simulink subsystem "EKF_IMU_GPS_3DoF"  (R2024b)
settings: Solver=VariableStepAuto  StartTime=0.0  StopTime=10.0  RelTol=1e-3
undefined symbols (not defined in the file or in its folder): filter_update_time, fractalcoef, lla_ref, u0, x0
libraries: sharedTrackingLibrary x1, sensorgpslib x1, mspsensorlib x1
settings Model: Creator=thatf  LastModifiedBy=thatf

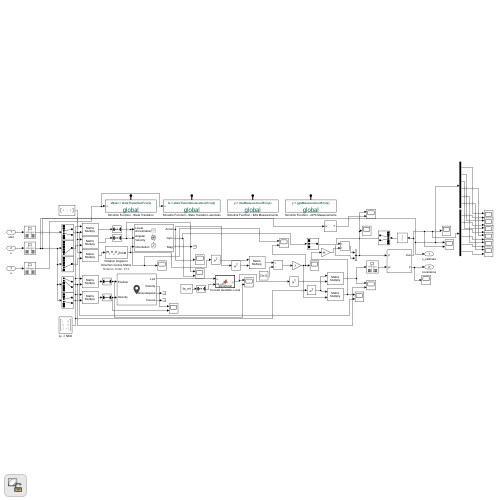
[thumbnail: Simulink's stored preview of the top-level diagram]
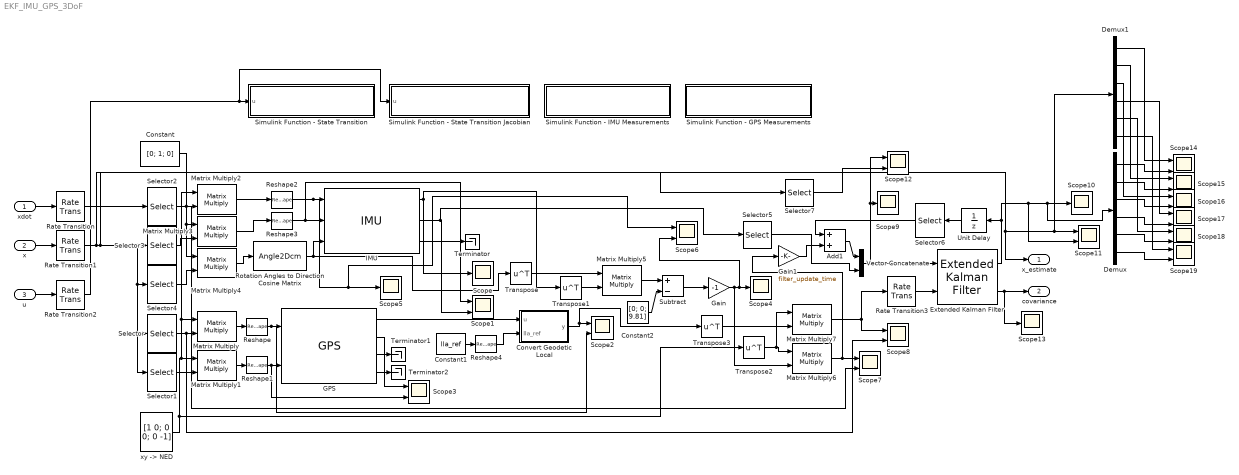
== system EKF_IMU_GPS_3DoF ==
  xdot : Inport
  x : Inport  Port=2
  u : Inport  Port=3
  Add1 : Sum
  Constant : Constant  Value=[0; 1; 0]
  Constant1 : Constant  Value=lla_ref
  Constant2 : Constant  Value=[0; 0; 9.81]
  Convert Geodetic Local : MATLAB Function  TreatAsAtomicUnit=on
  Demux : Demux  Outputs=6
  Demux1 : Demux  Outputs=6
  Extended Kalman Filter : sharedTrackingLibrary/Extended Kalman Filter  StateTransitionFcn=stateTransitionFcn  HasStateTransitionJacobianFcn=on  StateTransitionJacobianFcn=stateTransitionJacobianFcn  HasAdditiveProcessNoise=Additive  ProcessNoise=eye(6)*0.1  HasTimeVaryingProcessNoise=off  HasStateTransitionFcnExtraArgument=0  InitialState=x0'  InitialStateCovariance=eye(6)*0.1  MeasurementFcn1=imuMeasurementFcn  HasMeasurementJacobianFcn1=off  HasMeasurementEnablePort1=off  HasAdditiveMeasurementNoise1=Additive  MeasurementNoise1=[0.001;0.001;0.0001]  HasTimeVaryingMeasurementNoise1=off  HasMeasurementFcnExtraArgument1=0  HasMeasurementWrapping1=off  MeasurementFcn2=gpsMeasurementFcn  HasMeasurementJacobianFcn2=off  HasMeasurementEnablePort2=off  HasAdditiveMeasurementNoise2=Additive  MeasurementNoise2=[0.0005;.0001]  HasTimeVaryingMeasurementNoise2=off  HasMeasurementFcnExtraArgument2=0  HasMeasurementWrapping2=off  MeasurementFcn3=myMeasurementFcn  HasMeasurementJacobianFcn3=off  HasMeasurementEnablePort3=off  HasAdditiveMeasurementNoise3=Additive  MeasurementNoise3=1  HasTimeVaryingMeasurementNoise3=off  HasMeasurementFcnExtraArgument3=0  HasMeasurementWrapping3=off  MeasurementFcn4=myMeasurementFcn  HasMeasurementJacobianFcn4=off  HasMeasurementEnablePort4=off  HasAdditiveMeasurementNoise4=Additive  MeasurementNoise4=1  HasTimeVaryingMeasurementNoise4=off  HasMeasurementFcnExtraArgument4=0  HasMeasurementWrapping4=off  MeasurementFcn5=myMeasurementFcn  HasMeasurementJacobianFcn5=off  HasMeasurementEnablePort5=off  HasAdditiveMeasurementNoise5=Additive  MeasurementNoise5=1  HasTimeVaryingMeasurementNoise5=off  HasMeasurementFcnExtraArgument5=0  HasMeasurementWrapping5=off  EnableMultirate=on  StateTransitionFcnSampleTime=filter_update_time  MeasurementFcn1SampleTime=filter_update_time  MeasurementFcn2SampleTime=0.05  MeasurementFcn3SampleTime=1  MeasurementFcn4SampleTime=1  MeasurementFcn5SampleTime=1  UseCurrentEstimator=on  OutputStateCovariance=on  DataType=double  SampleTime=1  NumberOfMeasurements=2
  GPS : sensorgpslib/GPS  DispRefFrame=NED  PositionInputFormat=Local  ReferenceLocation=lla_ref  HorizontalPositionAccuracy=0.5  VerticalPositionAccuracy=1  VelocityAccuracy=0.1  DecayFactor=0.999  SeedDouble=67  SimulateUsing=Interpreted execution
  Gain : Gain  Gain=-1
  Gain1 : Gain  Gain=filter_update_time
  IMU : mspsensorlib/IMU  DispRefFrame=NED  TemperaturePort=off  Temperature=25  MagneticFieldPort=off  MagneticFieldNED=[ 27.5550, -2.4169, -16.0849 ]  MagneticFieldENU=[ -2.4169, 27.5550, 16.0849 ]  SeedDouble=67  SimulateUsing=Interpreted execution  AccelParamsMeasurementRange=Inf  AccelParamsResolution=0  AccelParamsConstantBias=[ 0, 0, 0 ]  AccelParamsAxesMisalignment=[ 100, 0, 0; 0, 100, 0; 0, 0, 100 ]  AccelParamsNoiseDensity=[ 0.01, 0.01, 0.01 ]  AccelParamsBiasInstability=[ 0, 0, 0 ]  AccelParamsBiasInstabilityNumerator=fractalcoef().Numerator  AccelParamsBiasInstabilityDenominator=fractalcoef().Denominator  AccelParamsRandomWalk=[ 0.01, 0.01, 0.01 ]  AccelParamsNoiseType=double-sided  AccelParamsTemperatureBias=[ 0, 0, 0 ]  AccelParamsTemperatureScaleFactor=[ 0, 0, 0 ]  GyroParamsMeasurementRange=Inf  GyroParamsResolution=0  GyroParamsConstantBias=[ 0, 0, 0 ]  GyroParamsAxesMisalignment=[ 100, 0, 0; 0, 100, 0; 0, 0, 100 ]  GyroParamsAccelerationBias=[ 0, 0, 0 ]  GyroParamsNoiseDensity=[ 0.0002, 0.0002, 0.0002 ]  GyroParamsBiasInstability=[ 0, 0, 0 ]  GyroParamsBiasInstabilityNumerator=fractalcoef().Numerator  GyroParamsBiasInstabilityDenominator=fractalcoef().Denominator  GyroParamsRandomWalk=[ 0.0002, 0.0002, 0.0002 ]  GyroParamsNoiseType=double-sided  GyroParamsTemperatureBias=[ 0, 0, 0 ]  GyroParamsTemperatureScaleFactor=[ 0, 0, 0 ]  MagParamsMeasurementRange=Inf  MagParamsResolution=0  MagParamsConstantBias=[ 0, 0, 0 ]  MagParamsAxesMisalignment=[ 100, 0, 0; 0, 100, 0; 0, 0, 100 ]  MagParamsNoiseDensity=[ 0, 0, 0 ]  MagParamsBiasInstability=[ 0, 0, 0 ]  MagParamsBiasInstabilityNumerator=fractalcoef().Numerator  MagParamsBiasInstabilityDenominator=fractalcoef().Denominator  MagParamsRandomWalk=[ 0, 0, 0 ]  MagParamsNoiseType=double-sided  MagParamsTemperatureBias=[ 0, 0, 0 ]  MagParamsTemperatureScaleFactor=[ 0, 0, 0 ]
  Matrix Multiply{,1..7} (8 alike) : Product  Multiplication=Matrix(*)
  Rate Transition : RateTransition  OutPortSampleTime=filter_update_time
  Rate Transition1 : RateTransition  InitialCondition=x0  OutPortSampleTime=filter_update_time
  Rate Transition2 : RateTransition  InitialCondition=u0  OutPortSampleTime=filter_update_time
  Rate Transition3 : RateTransition  InitialCondition=[x0(1), x0(2)]  OutPortSampleTime=0.05
  Reshape{,1..4} (5 alike) : Reshape  OutputDimensionality=Row vector (2-D)
  Rotation Angles to Direction Cosine Matrix : Angle2Dcm
      settings: AttributesFormatString=Rotation Order: %<rotationOrder>
  Scope{,4..5,9..10,13} (6 alike) : Scope
  Scope{1..3,6..8,11..12,14..19} (14 alike) : Scope  NumInputPorts=2
  Selector : Selector  InputPortWidth=6  IndexOptions=Index vector (dialog)  Indices=[1 2]  OutputSizes=1
  Selector1 : Selector  InputPortWidth=6  IndexOptions=Index vector (dialog)  Indices=[3 4]  OutputSizes=1
  Selector2 : Selector  InputPortWidth=6  IndexOptions=Index vector (dialog)  Indices=[3 4]  OutputSizes=1
  Selector3 : Selector  InputPortWidth=6  IndexOptions=Index vector (dialog)  Indices=[6]  OutputSizes=1
  Selector4 : Selector  InputPortWidth=6  IndexOptions=Index vector (dialog)  Indices=[5]  OutputSizes=1
  Selector5 : Selector  InputPortWidth=3  IndexOptions=Index vector (dialog)  Indices=[2]  OutputSizes=1
  Selector6 : Selector  InputPortWidth=6  IndexOptions=Index vector (dialog)  Indices=[3 4]  OutputSizes=1
  Selector7 : Selector  InputPortWidth=6  IndexOptions=Index vector (dialog)  Indices=[3 4 6]  OutputSizes=1
  Simulink Function - GPS Measurements : Subsystem  TreatAsAtomicUnit=on
  Simulink Function - IMU Measurements : Subsystem  TreatAsAtomicUnit=on
  Simulink Function - State Transition : Subsystem  TreatAsAtomicUnit=on
  Simulink Function - State Transition Jacobian : Subsystem  TreatAsAtomicUnit=on
  Subtract : Sum  Inputs=+-
  Terminator : Terminator
  Terminator1 : Terminator
  Terminator2 : Terminator
  Transpose{,1..3} (4 alike) : Math  Operator=transpose
  Unit Delay : UnitDelay  InitialCondition=x0  SampleTime=-1  HasFrameUpgradeWarning=on
  Vector Concatenate : Concatenate
  "xy -> NED" : Constant  Value=[1 0; 0 0; 0 -1]
  x_estimate : Outport
  covariance : Outport  Port=2
  wires:
  Constant2/1 -> Subtract/2
  Matrix Multiply5/1 -> Subtract/1
  Transpose2/1 -> Matrix Multiply6/1, Matrix Multiply7/1
  Selector/1 -> Matrix Multiply/2, Scope8/2
  Demux/3 -> Scope16/2
  Rate Transition1/1 -> Selector3/1, Selector4/1, Selector/1, Selector1/1, Scope11/1, Demux1/1, x_estimate/1, Selector7/1
  Add1/1 -> Vector Concatenate/1
  Matrix Multiply6/1 -> Scope7/1, Gain1/1
  Selector2/1 -> Matrix Multiply2/2, Scope7/2
  Constant/1 -> Matrix Multiply3/1, Matrix Multiply4/1
  Reshape3/1 -> IMU/2, Scope1/1
  Gain/1 -> Scope4/1, Scope6/2, Matrix Multiply6/2
  Selector4/1 -> Matrix Multiply4/2
  Subtract/1 -> Gain/1
  Demux/6 -> Scope19/2
  GPS/2 -> Scope3/1
  Selector7/1 -> Scope12/2
  Matrix Multiply2/1 -> Reshape2/1
  Transpose3/1 -> Matrix Multiply7/2
  Convert Geodetic Local/1(y) -> Scope2/1, Transpose3/1
  Unit Delay/1 -> Selector6/1
  Selector6/1 -> Add1/1
  Rotation Angles to Direction Cosine Matrix/1 -> IMU/3, Transpose/1
  Rate Transition2/1 -> Simulink Function - State Transition/1(u), Simulink Function - State Transition Jacobian/1(u)
  "xy -> NED"/1 -> Matrix Multiply1/1, Matrix Multiply2/1, Matrix Multiply/1, Transpose2/1
  Extended Kalman Filter/2 -> Scope13/1, covariance/1
  Reshape1/1 -> GPS/2, Scope3/2
  Rate Transition/1 -> Selector2/1
  Demux/5 -> Scope18/2
  Reshape2/1 -> IMU/1, Scope5/1, Scope6/1
  Matrix Multiply7/1 -> Rate Transition3/1, Scope8/1
  Demux1/3 -> Scope16/1
  Rate Transition3/1 -> Extended Kalman Filter/2
  Reshape4/1 -> Convert Geodetic Local/2(lla_ref)
  GPS/1 -> Convert Geodetic Local/1(u)
  IMU/2 -> Scope1/2, Selector5/1
  Demux/4 -> Scope17/2
  Demux1/2 -> Scope15/1
  Matrix Multiply/1 -> Reshape/1
  IMU/1 -> Transpose1/1, Scope/1
  Vector Concatenate/1 -> Extended Kalman Filter/1, Scope9/1, Scope12/1
  Matrix Multiply3/1 -> Reshape3/1
  Demux/2 -> Scope15/2
  GPS/3 -> Terminator1/1
  Transpose/1 -> Matrix Multiply5/1
  Transpose1/1 -> Matrix Multiply5/2
  Matrix Multiply1/1 -> Reshape1/1
  Matrix Multiply4/1 -> Rotation Angles to Direction Cosine Matrix/1
  Constant1/1 -> Reshape4/1
  Reshape/1 -> GPS/1, Scope2/2
  Selector5/1 -> Vector Concatenate/2
  Extended Kalman Filter/1 -> Scope10/1, Demux/1, Scope11/2, Unit Delay/1
  Selector1/1 -> Matrix Multiply1/2
  Selector3/1 -> Matrix Multiply3/2
  GPS/4 -> Terminator2/1
  Demux/1 -> Scope14/2
  Demux1/6 -> Scope19/1
  Demux1/4 -> Scope17/1
  Gain1/1 -> Add1/2
  Demux1/5 -> Scope18/1
  Demux1/1 -> Scope14/1
  IMU/3 -> Terminator/1
  xdot/1 -> Rate Transition/1
  x/1 -> Rate Transition1/1
  u/1 -> Rate Transition2/1

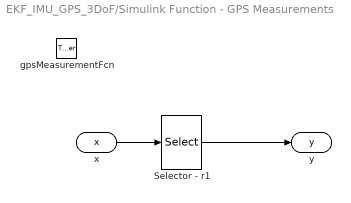
== system EKF_IMU_GPS_3DoF/Simulink Function - GPS Measurements ==
  gpsMeasurementFcn : TriggerPort  TriggerType=function-call  IsSimulinkFunction=on  FunctionName=gpsMeasurementFcn  VariantControl=Variant
  Selector - r1 : Selector  InputPortWidth=6  IndexOptions=Index vector (dialog)  Indices=[1, 2]  OutputSizes=1
  x : ArgIn  DisableCoverage=on  PortDimensions=6  ArgumentName=x
  y : ArgOut  DisableCoverage=on  PortDimensions=2  ArgumentName=y
  wires:
  x/1 -> Selector - r1/1
  Selector - r1/1 -> y/1

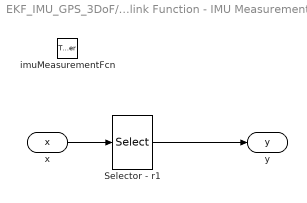
== system EKF_IMU_GPS_3DoF/Simulink Function - IMU Measurements ==
  imuMeasurementFcn : TriggerPort  TriggerType=function-call  IsSimulinkFunction=on  FunctionName=imuMeasurementFcn  VariantControl=Variant
  Selector - r1 : Selector  InputPortWidth=6  IndexOptions=Index vector (dialog)  Indices=[3, 4, 6]  OutputSizes=1
  x : ArgIn  DisableCoverage=on  PortDimensions=6  ArgumentName=x
  y : ArgOut  DisableCoverage=on  PortDimensions=3  ArgumentName=y
  wires:
  Selector - r1/1 -> y/1
  x/1 -> Selector - r1/1

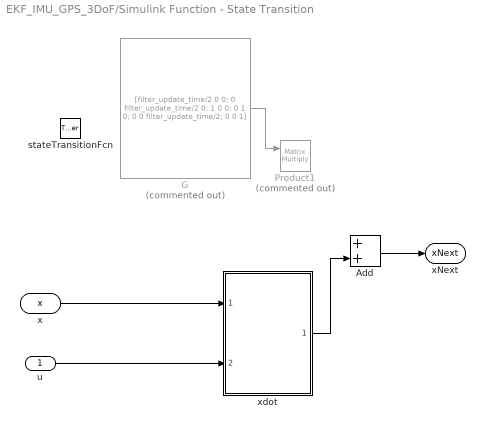
== system EKF_IMU_GPS_3DoF/Simulink Function - State Transition ==
  u : Inport
  stateTransitionFcn : TriggerPort  TriggerType=function-call  IsSimulinkFunction=on  FunctionName=stateTransitionFcn  VariantControl=Variant
  Add : Sum
  G : Constant  Commented=on  Value=[filter_update_time/2 0 0; 0 filter_update_time/2 0; 1 0 0; 0 1 0; 0 0 filter_update_time/2; 0 0 1]
  Product1 : Product  Commented=on  Multiplication=Matrix(*)
  xdot : Subsystem  ReferencedSubsystem=EoM_3DoF
  x : ArgIn  DisableCoverage=on  PortDimensions=6  ArgumentName=x
  xNext : ArgOut  DisableCoverage=on  PortDimensions=6  ArgumentName=xNext
  wires:
  xdot/1 -> Add/2
  Add/1 -> xNext/1
  u/1 -> xdot/2
  x/1 -> xdot/1
  G/1 -> Product1/1

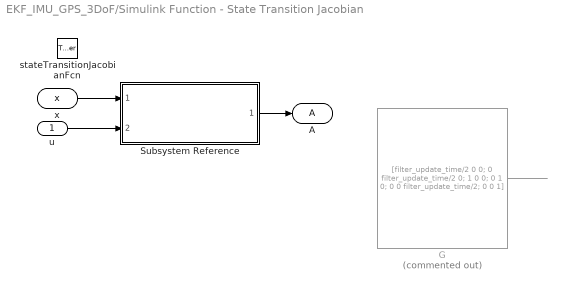
== system EKF_IMU_GPS_3DoF/Simulink Function - State Transition Jacobian ==
  u : Inport
  stateTransitionJacobianFcn : TriggerPort  TriggerType=function-call  IsSimulinkFunction=on  FunctionName=stateTransitionJacobianFcn  VariantControl=Variant
  G : Constant  Commented=on  Value=[filter_update_time/2 0 0; 0 filter_update_time/2 0; 1 0 0; 0 1 0; 0 0 filter_update_time/2; 0 0 1]
  Subsystem Reference : Subsystem  ReferencedSubsystem=JacobianX_3DoF
  x : ArgIn  DisableCoverage=on  PortDimensions=6  ArgumentName=x
  A : ArgOut  DisableCoverage=on  PortDimensions=[6 6]  ArgumentName=A
  wires:
  Subsystem Reference/1 -> A/1
  u/1 -> Subsystem Reference/2
  x/1 -> Subsystem Reference/1
  G/1 -> ?

== matlab function EKF_IMU_GPS_3DoF/Convert Geodetic Local ==
  data: u input; y output; lla_ref input
function y = geo2local(u, lla_ref)

y = lla2ned(u,lla_ref,"ellipsoid");

end
